simulink model "Exp2_bipolar_NRZ_RZ"  (R2020b)
settings: Solver=VariableStepAuto  StartTime=0.0  StopTime=10.0  RelTol=1e-3
libraries: simulink_extras x1, commrandsrc3 x1
settings Model: Creator=Mohit Akhouri  LastModifiedBy=Mohit Akhouri

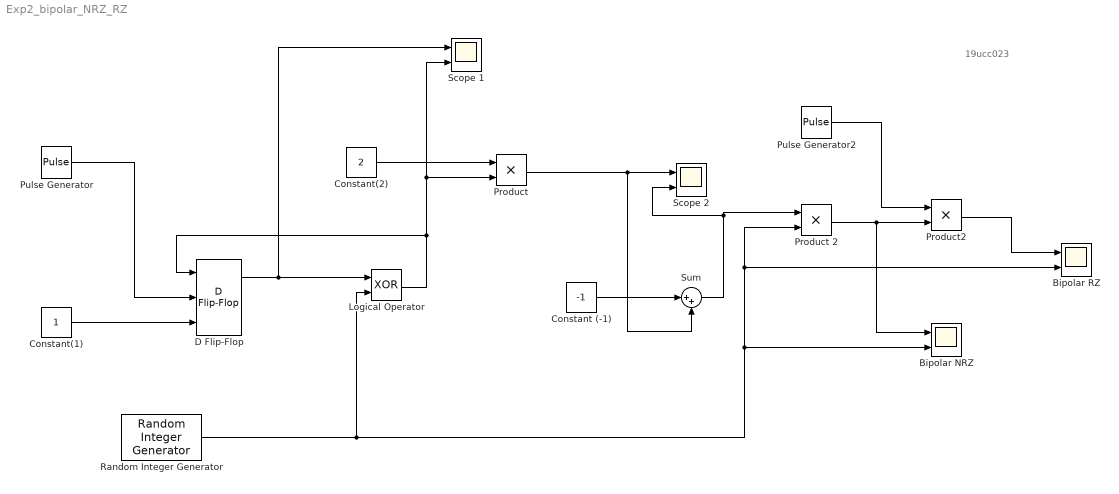
== system Exp2_bipolar_NRZ_RZ ==
  note: 19ucc023
  Bipolar NRZ : Scope  NumInputPorts=2
  Bipolar RZ : Scope  NumInputPorts=2
  Constant (-1) : Constant  Value=-1
  Constant(1) : Constant
  Constant(2) : Constant  Value=2
  D Flip-Flop : simulink_extras/Flip Flops/D Flip-Flop
  Logical Operator : Logic  Operator=XOR  AllPortsSameDT=off  OutDataTypeStr=boolean
  Product : Product
  Product 2 : Product
  Product2 : Product
  Pulse Generator : DiscretePulseGenerator  PulseType=Time based  Period=1  PulseWidth=50
  Pulse Generator2 : DiscretePulseGenerator  PulseType=Time based  Period=1  PulseWidth=50
  Random Integer Generator : commrandsrc3/Random Integer Generator  SetSize=2  SeedSource=Parameter  Seed=0  SampleTime=1  SamplesPerFrame=1  OutputDataType=double  SimulateUsing=Interpreted execution
  Scope 1 : Scope  NumInputPorts=2
  Scope 2 : Scope  NumInputPorts=2
  Sum : Sum  Inputs=|++
  wires:
  Constant(1)/1 -> D Flip-Flop/3
  Pulse Generator/1 -> D Flip-Flop/2
  D Flip-Flop/1 -> Scope 1/1, Logical Operator/1
  Logical Operator/1 -> D Flip-Flop/1, Product/2, Scope 1/2
  Constant(2)/1 -> Product/1
  Product/1 -> Sum/2, Scope 2/1
  Constant (-1)/1 -> Sum/1
  Random Integer Generator/1 -> Logical Operator/2, Bipolar NRZ/2, Bipolar RZ/2, Product 2/2
  Product2/1 -> Bipolar RZ/1
  Product 2/1 -> Bipolar NRZ/1, Product2/2
  Pulse Generator2/1 -> Product2/1
  Sum/1 -> Product 2/1, Scope 2/2
